simulink model "TriggerEdge4"  (R2020a)
settings: Solver=VariableStepAuto  StartTime=0.0  StopTime=2  RelTol=1e-3
settings Model: Creator=BEAR  LastModifiedBy=bzhan
settings DataIOCC: ReturnWorkspaceOutputs=off
settings DebuggingCC: ArithmeticOperatorsInVariantConditions=warning
settings SFSimCC: SimUseLocalCustomCode=off  CustomCodeUndefinedFunction=UseInterfaceOnly
settings RTWCC: RTWUseLocalCustomCode=off

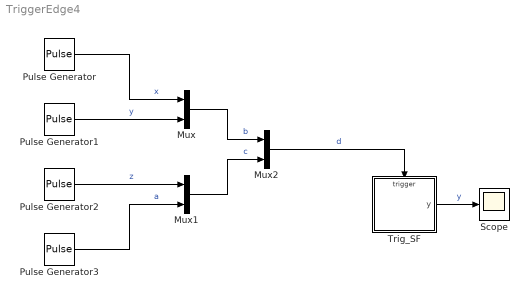
== system TriggerEdge4 ==
  Mux : Mux  Inputs=2
  Mux1 : Mux  Inputs=2
  Mux2 : Mux  Inputs=2
  Pulse Generator : DiscretePulseGenerator  PulseType=Time based  Period=1  PulseWidth=10  PhaseDelay=0.1
  Pulse Generator1 : DiscretePulseGenerator  PulseType=Time based  Period=1  PulseWidth=10  PhaseDelay=0.8
  Pulse Generator2 : DiscretePulseGenerator  PulseType=Time based  Period=1  PulseWidth=10  PhaseDelay=0.3
  Pulse Generator3 : DiscretePulseGenerator  PulseType=Time based  Period=1  PulseWidth=10  PhaseDelay=0.5
  Scope : Scope
  Trig_SF : Stateflow chart  TreatAsAtomicUnit=on
  wires:
  Pulse Generator/1 -> Mux/1  "x"
  Pulse Generator1/1 -> Mux/2  "y"
  Pulse Generator2/1 -> Mux1/1  "z"
  Pulse Generator3/1 -> Mux1/2  "a"
  Mux/1 -> Mux2/1  "b"
  Mux1/1 -> Mux2/2  "c"
  Mux2/1 -> Trig_SF/Trigger  "d"
  Trig_SF/1(y) -> Scope/1  "y"

== stateflow chart TriggerEdge4/Trig_SF ==
  settings: executeAtInitialization=1
  state A
  state B
    state B1
    state B2
    (default) -> B1
    B1 -> B2 : event2{y = 2;}
    B2 -> B1 : event3{y = 3;}
  (default) -> A
  A -> B : event{y = 0;}
  B -> A : event1{y = 1;}
  data: y output =-1
  events: event input RISING_EDGE_EVENT; event1 input RISING_EDGE_EVENT; event2 input RISING_EDGE_EVENT; event3 input RISING_EDGE_EVENT
